simulink model "LAB2_Norm_of_vector"  (R2022b)
settings: Solver=VariableStepAuto  StartTime=0.0  StopTime=10.0  RelTol=1e-3
values from neighbouring files (symbols this model uses):
  v = [0.1817 0.6198 -0.7634]    [LAB_02.m]
settings Model: Creator=ludov  LastModifiedBy=ludov

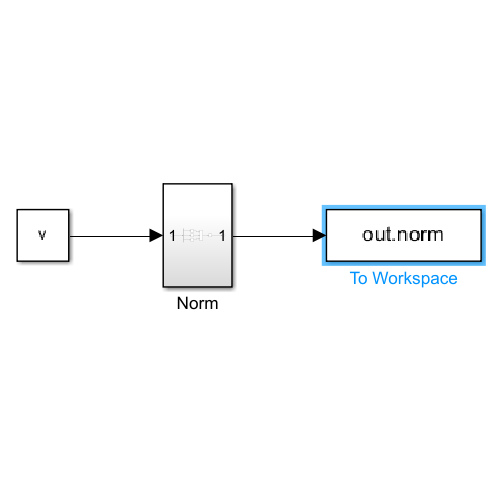
[thumbnail: Simulink's stored preview of the top-level diagram]
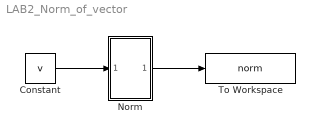
== system LAB2_Norm_of_vector ==
  Constant : Constant  Value=v
  Norm : Subsystem
  To Workspace : ToWorkspace  VariableName=norm  SaveFormat=Timeseries  SampleTime=-1
  wires:
  Constant/1 -> Norm/1(In1)
  Norm/1(Out1) -> To Workspace/1

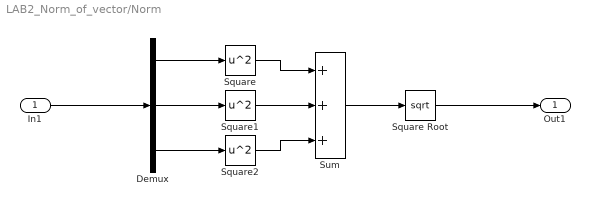
== system LAB2_Norm_of_vector/Norm ==
  In1 : Inport
  Demux : Demux  Outputs=3
  Square : Math  Operator=square
  Square Root : Sqrt
  Square1 : Math  Operator=square
  Square2 : Math  Operator=square
  Sum : Sum  Inputs=+++
  Out1 : Outport
  wires:
  Demux/3 -> Square2/1
  Sum/1 -> Square Root/1
  Demux/1 -> Square/1
  Square1/1 -> Sum/2
  Demux/2 -> Square1/1
  In1/1 -> Demux/1
  Square2/1 -> Sum/3
  Square/1 -> Sum/1
  Square Root/1 -> Out1/1
